simulink model "getDataFromXplane"  (R2022a)
settings: Solver=ode45  StartTime=0.0  StopTime=inf  RelTol=1e-3
libraries: etargetslib x1, sldrtlib x1, dspnetwork x1
settings Model: Creator=Flight Test Lab  LastModifiedBy=Ammar Abdurrauf
settings SolverCC: AlgebraicLoopSolver=TrustRegion
settings DataIOCC: SaveFormat=StructureWithTime  ReturnWorkspaceOutputs=off
settings OptimizationCC: LifeSpan=inf
settings DebuggingCC: UnconnectedInputMsg=warning  UnconnectedOutputMsg=warning  UnconnectedLineMsg=warning  SFExecutionAtInitializationDiag=none  SFMachineParentedDataDiag=warning  ArithmeticOperatorsInVariantConditions=warning
settings HardwareCC: ProdBitPerSizeT=32  ProdBitPerPtrDiffT=32  ProdWordSize=32  ProdHWDeviceType=Specified
settings SFSimCC: SimUseLocalCustomCode=off  CustomCodeUndefinedFunction=UseInterfaceOnly
settings RTWCC: RTWUseLocalCustomCode=off
settings CodeAppCC: StateflowObjectComments=on

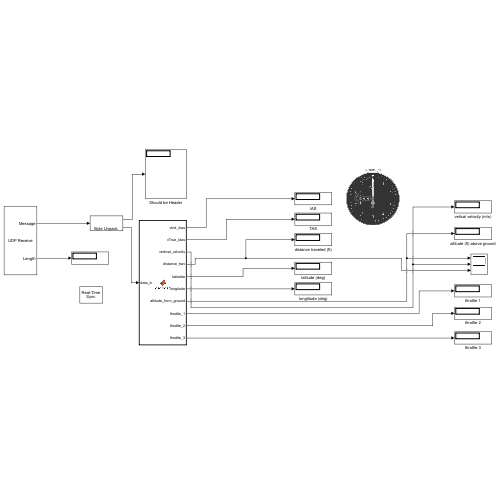
[thumbnail: Simulink's stored preview of the top-level diagram]
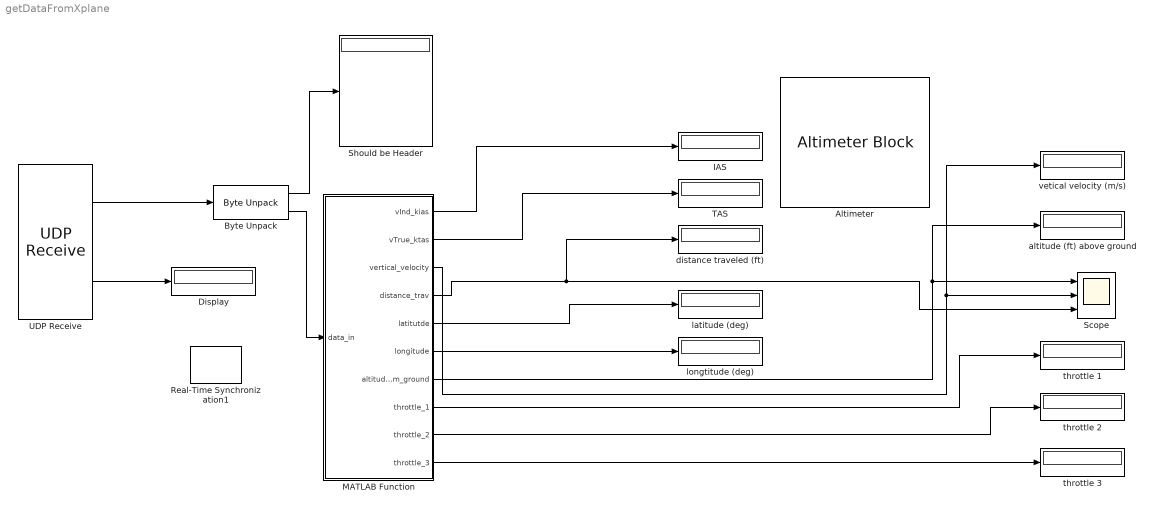
== system getDataFromXplane ==
  Altimeter : AltimeterBlock
  Byte Unpack : etargetslib/Byte Unpack  dimensions={5,[9,8]}  datatypes={'uint8','single'}  byteAlign=1
  Display : Display
  IAS : Display
  MATLAB Function : MATLAB Function  TreatAsAtomicUnit=on
  Real-Time Synchronization1 : sldrtlib/Real-Time Synchronization  SampleTime=0.000235  MaxMissedTicks=100  ShowMissedTicks=off  YieldWhenWaiting=off
  Scope : Scope  NumInputPorts=3
  Should be Header : Display
  TAS : Display
  UDP Receive : dspnetwork/UDP Receive  localURL='0.0.0.0'  localPort=49004  remoteURL='127.0.0.1'  remotePort=-1  recvBufferSize=8192  dims=293  signalDatatype=uint8  isComplex=off  isVarSize=off  showBlockingTime=off  blockingTime=0  sampletime=0.000235  blockPlatform=[]
  altitude (ft) above ground : Display
  distance traveled (ft) : Display
  latitude (deg) : Display
  longtitude (deg) : Display
  throttle 1 : Display
  throttle 2 : Display
  throttle 3 : Display
  vetical velocity (m/s) : Display
  wires:
  Byte Unpack/2 -> MATLAB Function/1(data_in)
  Byte Unpack/1 -> Should be Header/1
  UDP Receive/1 -> Byte Unpack/1
  MATLAB Function/3(vertical_velocity) -> Scope/2, vetical velocity (m/s)/1
  UDP Receive/2 -> Display/1
  MATLAB Function/2(vTrue_ktas) -> TAS/1
  MATLAB Function/1(vInd_kias) -> IAS/1
  MATLAB Function/4(distance_trav) -> Scope/3, distance traveled (ft)/1
  MATLAB Function/5(latitutde) -> latitude (deg)/1
  MATLAB Function/6(longitude) -> longtitude (deg)/1
  MATLAB Function/7(altitude_from_ground) -> Scope/1, altitude (ft) above ground/1
  MATLAB Function/8(throttle_1) -> throttle 1/1
  MATLAB Function/9(throttle_2) -> throttle 2/1
  MATLAB Function/10(throttle_3) -> throttle 3/1

== matlab function getDataFromXplane/MATLAB Function ==
  data: data_in input; vInd_kias output; vTrue_ktas output; vertical_velocity output; distance_trav output; latitutde output; longitude output; altitude_from_ground output; throttle_1 output; throttle_2 output; throttle_3 output
function [vInd_kias,vTrue_ktas,...
    vertical_velocity, distance_trav,...
    latitutde, longitude, altitude_from_ground,...
    throttle_1, throttle_2, throttle_3] = decoder(data_in)
 
 vInd_kias = data_in(2,1);
 vTrue_ktas = data_in(4,1);
 latitutde= data_in(2,2);
 longitude= data_in(3,2);
 altitude_from_ground= data_in(5,2);
 vertical_velocity= data_in(6,3);
 distance_trav= data_in(8,3);
 throttle_1 = data_in(2, 4);
 throttle_2 = data_in(3, 4);
 throttle_3 = data_in(4, 4);
end
